simulink library "xrbsComm_r3"  (Simulink 5.1)
libraries: xbsIndex_r3 x775, xrbsComm_r3 x1
(part 1 of 6)
settings Model: Creator=singhj  LastModifiedBy=annr  ProdHWDeviceType=Microprocessor

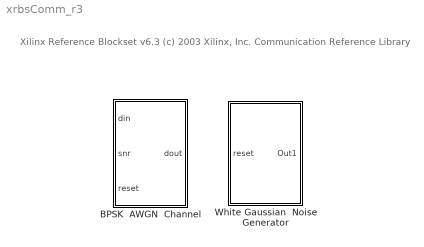
== system xrbsComm_r3 ==
  note: Xilinx Reference Blockset v6.3
      | (c) 2003  Xilinx, Inc.
      |
      | Communication Reference Library
  BPSK  AWGN  Channel : Subsystem  mask(BPSK AWGN Channel){seed=510}
      mask prompts: seed "Decimal Seed Value"
      mask help: Binary Phase Shift Keying Additive White Gaussian Noise Channel. Adds scaled white Gaussian nose to an input signal.
      mask init:
      | [bg,fg] = xlcmap('XBlock',0);
      | iPos = get_param(gcb,'Position');
      | iWidth=iPos(3)-iPos(1); iHeight=iPos(4)-iPos(2);
      | iCx=iWidth/2;
      | iCy=iHeight/2;
      | [logoX, logoY] = xlogo(iPos);
      mask Help:
      | web(xldoclink('BPSK
      | AWGN
      | Channel'));
      mask Display:
      | patch([0 iWidth iWidth 0],[0 0 iHeight iHeight] , bg);
      | patch(logoX,logoY , fg);
      | port_label('input',1,'din');
      | port_label('input',2,'snr');
      | port_label('input',3,'reset');
      | port_label('output',1,'dout');
      | plot([0 0 iWidth iWidth 0], [0 iHeight iHeight 0 0]);
  White Gaussian  Noise Generator : Subsystem  mask(White Gaussian Noise Generator){seed=512}
      mask help: White Gaussian Noise Generator. Generates white Gaussian noise using a combination of the Box-Muller algorithm and the central limit theorem.
      mask init:
      | old_seed = rand('seed');
      | rand('seed',seed);
      | init1 = [dec2hex(floor(rand*16)) dec2hex(floor(rand*16)) dec2hex(floor(rand*16)) ...
      | 		dec2hex(floor(rand*16)) dec2hex(floor(rand*16)) dec2hex(floor(rand*16)) ...
      | 		dec2hex(floor(rand*16)) dec2hex(floor(rand*16)) dec2hex(floor(rand*16)) ...
      | 		dec2hex(floor(rand*16)) dec2hex(floor(rand*16)) dec2hex(floor(rand*16))];
      | seed1 = hex2dec(init1);
      | init2 = [dec2hex(floor(rand*16)) dec2hex(floor(rand*16)) dec2hex(floor(rand*16)) ...
      | 		dec2hex(floor(rand*16)) dec2hex(floor(rand*16)) dec2hex(floor(rand*16)) ...
      | 		dec2hex(floor(rand*16)) dec2hex(floor(rand*16)) dec2hex(floor(rand*16)) ...
      | 		dec2hex(floor(rand*16)) dec2hex(floor(rand*16)) dec2hex(floor(rand*16))];
      | seed2 = hex2dec(init2);
      | init3 = [dec2hex(floor(rand*16)) dec2hex(floor(rand*16)) dec2hex(floor(rand*16)) ...
      | 		dec2hex(floor(rand*16)) dec2hex(floor(rand*16)) dec2hex(floor(rand*16)) ...
      | 		dec2hex(floor(rand*16)) dec2hex(floor(rand*16)) dec2hex(floor(rand*16)) ...
      | 		dec2hex(floor(rand*16)) dec2hex(floor(rand*16)) dec2hex(floor(rand*16))];
      | seed3 = hex2dec(init3);
      | init4 = [dec2hex(floor(rand*16)) dec2hex(floor(rand*16)) dec2hex(floor(rand*16)) ...
      | 		dec2hex(floor(rand*16)) dec2hex(floor(rand*16)) dec2hex(floor(rand*16)) ...
      | 		dec2hex(floor(rand*16)) dec2hex(floor(rand*16)) dec2hex(floor(rand*16)) ...
      | 		dec2hex(floor(rand*16)) dec2hex(floor(rand*16)) dec2hex(floor(rand*16))];
      | seed4 = hex2dec(init4);
      | rand('seed',old_seed);
      | 
      | 
      | [bg,fg] = xlcmap('XBlock',0);
      | iPos = get_param(gcb,'Position');
      | iWidth=iPos(3)-iPos(1); iHeight=iPos(4)-iPos(2);
      | iCx=iWidth/2;
      | iCy=iHeight/2;
      | [logoX, logoY] = xlogo(iPos);
      mask Help: web(xlhtmldoclink('White Gaussian  Noise Generator'));
      mask Display:
      | patch([0 iWidth iWidth 0],[0 0 iHeight iHeight] , bg);
      | patch(logoX,logoY , fg);
      | port_label('input',1,'reset');
      | port_label('output',1,'noise');
      | plot([0 0 iWidth iWidth 0], [0 iHeight iHeight 0 0]);

== system xrbsComm_r3/BPSK  AWGN  Channel ==
  note: The WGNG block generates a probability density function (PDF) that is Gaussian to within .2% for
      | 4.8 standard deviations from the mean.  The PDF is scaled based on the value of the signal to noise
      | ratio to achieve the desired noise variance.  The SNR input is defined as (Eb/No) in dB for uncoded BPSK
      | with unit symbol energy (Es = 1).  If the SNR input is of type UFix8_4, the valid range is from 0.0 to 15.9375
      | in steps of 0.0625dB.  To use the AWGN in a system with coding and/or to use the core with different
      | modulation formats, it is necessary to adjust the SNR value to accommodate the difference in spectral
      | efficiency.  If we have BPSK modulation with rate 1/2 coding and keep Es = 1and No constant, then Eb = 2
      | and Eb/No = SNR + 3 dB.  If we have uncoded QPSK modulation with I = +/-1 and Q = +/-1 and add
      | independent noise sequences, then each channel looks like and independent BPSK channel and the
      | Eb/No = SNR.  If we then add rate 1/2 coding to the QPSK case, we have Eb/No = SNR + 3 dB.
      |
      | For more information see:
      |
      | [1] A. Ghazel, E. Boutillon, J. L. Danger, G. Gulak and H. Laamari, "Design and Performance Analysis of a
      | High Speed AWGN Communication Channel Emulator" IEEE PACRIM Conference, Victoria, B. C., Aug.
      | 2001.
      | [2] Xilinx Data Sheet: Additive White Gaussian Noise (AWGN) Core v1.0, Xilinx, Inc. October 2002
  din : Inport
  snr : Inport  Port=2
  reset : Inport  Port=3
  AddSub : xbsIndex_r3/AddSub  mode=Addition  precision=Full  arith_type=Unsigned  n_bits=8  bin_pt=2  quantization=Truncate  overflow=Wrap  latency=1  explicit_period=off  period=1  use_carryin=off  use_carryout=off  en=off  dbl_ovrd=off  show_param=off  use_core=on  pipeline=off  use_rpm=off  gen_core=on
      settings: xl_area=[0, 0, 0, 0, 0, 0, 0]
  Constant1 : xbsIndex_r3/Constant  const=1  arith_type="Signed  (2's comp)"  n_bits=2  bin_pt=0  explicit_period=off  period=1  dbl_ovrd=off
  Constant2 : xbsIndex_r3/Constant  const=-1  arith_type="Signed  (2's comp)"  n_bits=2  bin_pt=0  explicit_period=off  period=1  dbl_ovrd=off
  Convert : xbsIndex_r3/Convert  arith_type="Signed  (2's comp)"  n_bits=16  bin_pt=11  quantization="Round  (unbiased: +/- Inf)"  overflow=Wrap  latency=2  explicit_period=off  period=1  dbl_ovrd=off  show_param=off  inserted_by_tool=off
      settings: xl_area=[0, 0, 0, 0, 0, 0, 0]
  Delay : xbsIndex_r3/Delay  latency=14  reg_retiming=off  explicit_period=off  period=1  en=off  accept_only_valid=off  init_zero=on  dbl_ovrd=off  show_param=off
      settings: xl_area=[0, 0, 0, 0, 0, 0, 0]
  Input  Conversion : Subsystem
  Mult : xbsIndex_r3/Mult  precision=Full  arith_type="Signed  (2's comp)"  n_bits=8  bin_pt=2  quantization=Truncate  overflow=Wrap  latency=2  explicit_period=off  period=1  en=off  dbl_ovrd=off  show_param=off  mult_type=Parallel  oversample=2  use_embedded=on  pipeline=off  use_rpm=off  placement_style=Rectangular Shape  gen_core=on
      settings: xl_area=[0, 0, 0, 0, 0, 0, 0]
  Mux : xbsIndex_r3/Mux  inputs=2  precision=Full  arith_type="Signed  (2's comp)"  n_bits=8  bin_pt=2  quantization=Truncate  overflow=Wrap  latency=0  explicit_period=off  period=-1  en=off  dbl_ovrd=off  show_param=off  mux_type=off  use_rpm=off  gen_core=on
      settings: xl_area=[0, 0, 0, 0, 0, 0, 0]
  ROM : xbsIndex_r3/ROM  depth=256  initVector=((2*10.^(0.1*(([0:255]/10) - 0.6*floor([0:255]/16) ))).^(-0.5))*1.0023  arith_type=Unsigned  n_bits=15  bin_pt=15  latency=1  init_zero=on  explicit_period=off  period=1  rst=off  init_reg=0  en=off  dbl_ovrd=off  show_param=off  distributed_mem=off  use_rpm=off  gen_core=on
      settings: xl_area=[0, 0, 0, 0, 0, 0, 0]
  White Gaussian  Noise Generator : xrbsComm_r3/White Gaussian  Noise Generator  seed=512
  dout : Outport
  wires:
  reset/1 -> White Gaussian  Noise Generator/1
  Delay/1 -> AddSub/1
  Convert/1 -> AddSub/2
  White Gaussian  Noise Generator/1 -> Mult/2
  din/1 -> Mux/1
  snr/1 -> Input  Conversion/1(" ")
  Mult/1 -> Convert/1
  ROM/1 -> Mult/1
  AddSub/1 -> dout/1
  Input  Conversion/1(conv) -> ROM/1
  Constant1/1 -> Mux/2
  Constant2/1 -> Mux/3
  Mux/1 -> Delay/1

== system xrbsComm_r3/White Gaussian  Noise Generator ==
  note: The WGNG generates white Gaussian noise using a combination of the Box-Muller algorithm and the Central Limit Theorem
      | following the general approach described in [1].   The Box-Muller algorithm generates a unit normal random variable via a
      | transformation of two independent random variables that are uniformly distributed over [0,1].  This is accomplished by storing
      | Box-Muller function values in ROMs and addressing them with uniform random variables.  The uniform random variables are
      | produced by multiple-bit leap-forward LFSRs.  A standard LFSR generates one output per clock cycle.  K-bit leap-forward LFSRs
      | are able to generate k outputs in a single cycle.  For example, a 4-bit leap-forward LFSR outputs a discrete uniform random
      | variable between 0 and 15.  A portion of the 48-bit block parameter seed initializes each LFSR allowing customization.  The
      | outputs of four parallel Box-Muller subsystems are averaged to obtain a probability density function (PDF) that is Gaussian.
      | The overall latency of the WGNG is 10 clock cycles.  The output port noise is a 12 bit signed number with 7 bits after the binary
      | point.
      |
      | [1] A. Ghazel, E. Boutillon, J. L. Danger, G. Gulak and H. Laamari, "Design and Performance Analysis of a
      | High Speed AWGN Communication Channel Emulator" IEEE PACRIM Conference, Victoria, B. C., Aug. 2001.
  " reset" : Inport
  AddSub : xbsIndex_r3/AddSub  mode=Addition  precision=Full  arith_type=Unsigned  n_bits=8  bin_pt=2  quantization=Truncate  overflow=Wrap  latency=1  explicit_period=off  period=1  use_carryin=off  use_carryout=off  en=off  dbl_ovrd=off  show_param=off  use_core=on  pipeline=off  use_rpm=off  gen_core=on
      settings: xl_area=[0, 0, 0, 0, 0, 0, 0]
  AddSub1 : xbsIndex_r3/AddSub  mode=Addition  precision=Full  arith_type=Unsigned  n_bits=8  bin_pt=2  quantization=Truncate  overflow=Wrap  latency=1  explicit_period=off  period=1  use_carryin=off  use_carryout=off  en=off  dbl_ovrd=off  show_param=off  use_core=on  pipeline=off  use_rpm=off  gen_core=on
      settings: xl_area=[0, 0, 0, 0, 0, 0, 0]
  AddSub2 : xbsIndex_r3/AddSub  mode=Addition  precision=Full  arith_type=Unsigned  n_bits=8  bin_pt=2  quantization=Truncate  overflow=Wrap  latency=1  explicit_period=off  period=1  use_carryin=off  use_carryout=off  en=off  dbl_ovrd=off  show_param=off  use_core=on  pipeline=off  use_rpm=off  gen_core=on
      settings: xl_area=[0, 0, 0, 0, 0, 0, 0]
  Box-Muller1 : Subsystem  mask(Box-Muller){f_init1=bitget(seed1, 17:-1:1), f_init2=bitget(seed1, 25:-1:1), f_init3=bitget(seed1, 29:-1:1), f_init4=bitget(seed1, 31:-1:1), f_init5=bitget(seed1, 41:-1:1), g_init=bitget(seed1, 47:-1:1)}
      mask prompts: f_init1 "f_init1(17:1)"; f_init2 "f_init2(25:1)"; f_init3 "f_init3(29:1)"; f_init4 "f_init4(31:1)"; f_init5 "f_init5(41:1)"; g_init "g_init(47:1)"
  Box-Muller2 : Subsystem  mask(Box-Muller){f_init1=bitget(seed2, 17:-1:1), f_init2=bitget(seed2, 25:-1:1), f_init3=bitget(seed2, 29:-1:1), f_init4=bitget(seed2, 31:-1:1), f_init5=bitget(seed2, 41:-1:1), g_init=bitget(seed2, 47:-1:1)}
      mask prompts: f_init1 "f_init1(17:1)"; f_init2 "f_init2(25:1)"; f_init3 "f_init3(29:1)"; f_init4 "f_init4(31:1)"; f_init5 "f_init5(41:1)"; g_init "g_init(47:1)"
  Box-Muller3 : Subsystem  mask(Box-Muller){f_init1=bitget(seed3, 17:-1:1), f_init2=bitget(seed3, 25:-1:1), f_init3=bitget(seed3, 29:-1:1), f_init4=bitget(seed3, 31:-1:1), f_init5=bitget(seed3, 41:-1:1), g_init=bitget(seed3,47:-1:1)}
      mask prompts: f_init1 "f_init1(17:1)"; f_init2 "f_init2(25:1)"; f_init3 "f_init3(29:1)"; f_init4 "f_init4(31:1)"; f_init5 "f_init5(41:1)"; g_init "g_init(47:1)"
  Box-Muller4 : Subsystem  mask(Box-Muller){f_init1=bitget(seed4, 17:-1:1), f_init2=bitget(seed4, 25:-1:1), f_init3=bitget(seed4, 29:-1:1), f_init4=bitget(seed4, 31:-1:1), f_init5=bitget(seed4, 41:-1:1), g_init=bitget(seed4, 47:-1:1)}
      mask prompts: f_init1 "f_init1(17:1)"; f_init2 "f_init2(25:1)"; f_init3 "f_init3(29:1)"; f_init4 "f_init4(31:1)"; f_init5 "f_init5(41:1)"; g_init "g_init(47:1)"
  Reinterpret : xbsIndex_r3/Reinterpret  force_arith_type=off  arith_type=Unsigned  force_bin_pt=on  bin_pt=7  force_valid=on
  Out1 : Outport
  wires:
  " reset"/1 -> Box-Muller3/1(reset), Box-Muller4/1(reset), Box-Muller2/1(reset), Box-Muller1/1(" reset")
  Reinterpret/1 -> Out1/1
  Box-Muller4/1(bm) -> AddSub1/2
  Box-Muller3/1(bm) -> AddSub1/1
  Box-Muller2/1(bm) -> AddSub/2
  Box-Muller1/1(bm) -> AddSub/1
  AddSub2/1 -> Reinterpret/1
  AddSub1/1 -> AddSub2/2
  AddSub/1 -> AddSub2/1

== system xrbsComm_r3/BPSK  AWGN  Channel/Input  Conversion ==
  " " : Inport
  AddSub1 : xbsIndex_r3/AddSub  mode=Addition  precision=User Defined  arith_type=Unsigned  n_bits=8  bin_pt=0  quantization=Truncate  overflow=Wrap  latency=0  explicit_period=off  period=1  en=off  dbl_ovrd=off  use_core=on  gen_core=on  pipeline=off  use_rpm=off
      settings: xl_area=[0, 0, 0, 0, 0, 0, 0]
  CMult : xbsIndex_r3/CMult  const=16  const_n_bits=5  const_bin_pt=0  precision=Full  arith_type="Signed  (2's comp)"  n_bits=8  bin_pt=6  quantization="Round  (unbiased: +/- Inf)"  overflow=Wrap  mult_type=Parallel  mem_type=Distributed RAM  pipeline=off  latency=0  explicit_period=off  period=1  en=off  dbl_ovrd=off  oversample=2  gen_core=on  use_rpm=off  placement_style=Rectangular Shape
      settings: xl_area=[0, 0, 0, 0, 0, 0, 0]
  CMult1 : xbsIndex_r3/CMult  const=10  const_n_bits=4  const_bin_pt=0  precision=Full  arith_type="Signed  (2's comp)"  n_bits=8  bin_pt=6  quantization="Round  (unbiased: +/- Inf)"  overflow=Wrap  mult_type=Parallel  mem_type=Distributed RAM  pipeline=off  latency=0  explicit_period=off  period=1  en=off  dbl_ovrd=off  oversample=2  gen_core=on  use_rpm=off  placement_style=Rectangular Shape
      settings: xl_area=[0, 0, 0, 0, 0, 0, 0]
  Shift : xbsIndex_r3/Shift  shift_dir=Right  shift_bits=4  precision=User Defined  arith_type=Unsigned  n_bits=4  bin_pt=0  quantization=Truncate  overflow=Wrap  latency=0  explicit_period=off  period=1  en=off  dbl_ovrd=off
      settings: xl_area=[0, 0, 0, 0, 0, 0, 0]
  Slice : xbsIndex_r3/Slice  mode=Upper Bit Location + Width  nbits=4  bit1=0  base1=MSB of Input  bit0=0  base0=LSB of Input  boolean_output=off  explicit_period=off  period=1  dbl_ovrd=off
  Slice1 : xbsIndex_r3/Slice  mode=Lower Bit Location + Width  nbits=4  bit1=0  base1=MSB of Input  bit0=0  base0=LSB of Input  boolean_output=off  explicit_period=off  period=1  dbl_ovrd=off
  conv : Outport
  wires:
  Slice/1 -> CMult/1
  Slice1/1 -> CMult1/1
  AddSub1/1 -> conv/1
  CMult/1 -> AddSub1/1
  " "/1 -> Slice/1, Slice1/1
  CMult1/1 -> Shift/1
  Shift/1 -> AddSub1/2

== system xrbsComm_r3/White Gaussian  Noise Generator/Box-Muller1 ==
  " reset" : Inport
  Convert : xbsIndex_r3/Convert  arith_type="Signed  (2's comp)"  n_bits=10  bin_pt=6  quantization="Round  (unbiased: +/- Inf)"  overflow=Wrap  latency=2  explicit_period=off  period=1  dbl_ovrd=off  inserted_by_tool=off
      settings: xl_area=[0, 0, 0, 0, 0, 0, 0]
  Mult : xbsIndex_r3/Mult  precision=Full  arith_type="Signed  (2's comp)"  n_bits=20  bin_pt=0  quantization="Round  (unbiased: +/- Inf)"  overflow=Wrap  mult_type=Parallel  use_embedded=on  pipeline=on  latency=2  explicit_period=off  period=1  en=off  dbl_ovrd=off  oversample=2  gen_core=on  use_rpm=off  placement_style=Rectangular Shape
      settings: xl_area=[0, 0, 0, 0, 0, 0, 0]
  f : Subsystem  mask(f_rom){init1=f_init1, init2=f_init2, init3=f_init3, init4=f_init4, init5=f_init5}
      mask prompts: init1 "init1(17:1)"; init2 "init2(25:1)"; init3 "init3(29:1)"; init4 "init4(31:1)"; init5 "init5(41:1)"
  g : Subsystem  mask{init=g_init}
      mask prompts: init "g_init(47:1)"
  bm : Outport
  wires:
  g/1(g(s')) -> Mult/2
  f/1(f(s')) -> Mult/1
  Mult/1 -> Convert/1
  Convert/1 -> bm/1
  " reset"/1 -> f/1("reset "), g/1(reset)

== system xrbsComm_r3/White Gaussian  Noise Generator/Box-Muller2 ==
  reset : Inport
  Convert : xbsIndex_r3/Convert  arith_type="Signed  (2's comp)"  n_bits=10  bin_pt=6  quantization="Round  (unbiased: +/- Inf)"  overflow=Wrap  latency=2  explicit_period=off  period=1  dbl_ovrd=off  inserted_by_tool=off
      settings: xl_area=[0, 0, 0, 0, 0, 0, 0]
  Mult : xbsIndex_r3/Mult  precision=Full  arith_type="Signed  (2's comp)"  n_bits=20  bin_pt=0  quantization="Round  (unbiased: +/- Inf)"  overflow=Wrap  mult_type=Parallel  use_embedded=on  pipeline=on  latency=2  explicit_period=off  period=1  en=off  dbl_ovrd=off  oversample=2  gen_core=on  use_rpm=off  placement_style=Rectangular Shape
      settings: xl_area=[0, 0, 0, 0, 0, 0, 0]
  fr1 : Subsystem  mask(f_rom){init1=f_init1, init2=f_init2, init3=f_init3, init4=f_init4, init5=f_init5}
      mask prompts: init1 "init1(17:1)"; init2 "init2(25:1)"; init3 "init3(29:1)"; init4 "init4(31:1)"; init5 "init5(41:1)"
  g2 : Subsystem  mask{init=g_init}
      mask prompts: init "g_init(47:1)"
  bm : Outport
  wires:
  g2/1(g(s')) -> Mult/2
  Mult/1 -> Convert/1
  Convert/1 -> bm/1
  reset/1 -> fr1/1(reset), g2/1(reset)
  fr1/1(f(s')) -> Mult/1

== system xrbsComm_r3/White Gaussian  Noise Generator/Box-Muller3 ==
  reset : Inport
  Convert : xbsIndex_r3/Convert  arith_type="Signed  (2's comp)"  n_bits=10  bin_pt=6  quantization="Round  (unbiased: +/- Inf)"  overflow=Wrap  latency=2  explicit_period=off  period=1  dbl_ovrd=off  inserted_by_tool=off
      settings: xl_area=[0, 0, 0, 0, 0, 0, 0]
  Mult : xbsIndex_r3/Mult  precision=Full  arith_type="Signed  (2's comp)"  n_bits=20  bin_pt=0  quantization="Round  (unbiased: +/- Inf)"  overflow=Wrap  mult_type=Parallel  use_embedded=on  pipeline=on  latency=2  explicit_period=off  period=1  en=off  dbl_ovrd=off  oversample=2  gen_core=on  use_rpm=off  placement_style=Rectangular Shape
      settings: xl_area=[0, 0, 0, 0, 0, 0, 0]
  fr1 : Subsystem  mask(f_rom){init1=f_init1, init2=f_init2, init3=f_init3, init4=f_init4, init5=f_init5}
      mask prompts: init1 "init1(17:1)"; init2 "init2(25:1)"; init3 "init3(29:1)"; init4 "init4(31:1)"; init5 "init5(41:1)"
  g2 : Subsystem  mask{init=g_init}
      mask prompts: init "g_init(47:1)"
  bm : Outport
  wires:
  g2/1(g(s')) -> Mult/2
  fr1/1(f(s')) -> Mult/1
  Mult/1 -> Convert/1
  Convert/1 -> bm/1
  reset/1 -> fr1/1(reset), g2/1(reset)

== system xrbsComm_r3/White Gaussian  Noise Generator/Box-Muller4 ==
  reset : Inport
  Convert : xbsIndex_r3/Convert  arith_type="Signed  (2's comp)"  n_bits=10  bin_pt=6  quantization="Round  (unbiased: +/- Inf)"  overflow=Wrap  latency=2  explicit_period=off  period=1  dbl_ovrd=off  inserted_by_tool=off
      settings: xl_area=[0, 0, 0, 0, 0, 0, 0]
  Mult : xbsIndex_r3/Mult  precision=Full  arith_type="Signed  (2's comp)"  n_bits=20  bin_pt=0  quantization="Round  (unbiased: +/- Inf)"  overflow=Wrap  mult_type=Parallel  use_embedded=on  pipeline=on  latency=2  explicit_period=off  period=1  en=off  dbl_ovrd=off  oversample=2  gen_core=on  use_rpm=off  placement_style=Rectangular Shape
      settings: xl_area=[0, 0, 0, 0, 0, 0, 0]
  fr1 : Subsystem  mask(f_rom){init1=f_init1, init2=f_init2, init3=f_init3, init4=f_init4, init5=f_init5}
      mask prompts: init1 "init1(17:1)"; init2 "init2(25:1)"; init3 "init3(29:1)"; init4 "init4(31:1)"; init5 "init5(41:1)"
  g2 : Subsystem  mask{init=g_init}
      mask prompts: init "g_init(47:1)"
  bm : Outport
  wires:
  reset/1 -> g2/1(reset), fr1/1(reset)
  g2/1(g(s')) -> Mult/2
  fr1/1(f(s')) -> Mult/1
  Mult/1 -> Convert/1
  Convert/1 -> bm/1

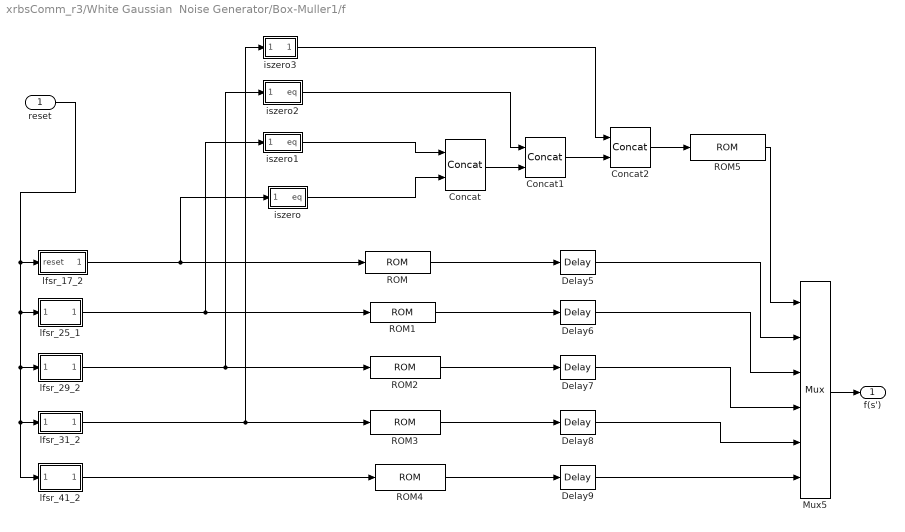
== system xrbsComm_r3/White Gaussian  Noise Generator/Box-Muller1/f ==
  "reset " : Inport
  Concat : xbsIndex_r3/Concat  explicit_period=off  period=1  dbl_ovrd=off
  Concat1 : xbsIndex_r3/Concat  explicit_period=off  period=1  dbl_ovrd=off
  Concat2 : xbsIndex_r3/Concat  explicit_period=off  period=1  dbl_ovrd=off
  Delay{5..9} (5 alike) : xbsIndex_r3/Delay  latency=2  explicit_period=off  period=1  en=off  accept_only_valid=off  init_zero=on  dbl_ovrd=off
      settings: xl_area=[0, 0, 0, 0, 0, 0, 0]
  Mux5 : xbsIndex_r3/Mux  inputs=5  precision=Full  arith_type="Signed  (2's comp)"  n_bits=10  bin_pt=0  quantization="Round  (unbiased: +/- Inf)"  overflow=Wrap  latency=1  mux_type=off  explicit_period=off  period=1  en=off  dbl_ovrd=off  gen_core=on  use_rpm=off
      settings: xl_area=[0, 0, 0, 0, 0, 0, 0]
  ROM : xbsIndex_r3/ROM  depth=16  initVector=sqrt(-log( ((0:15)+0.51)'*(2.^(-1.*4)) ))  arith_type=Unsigned  n_bits=9  bin_pt=7  latency=1  distributed_mem=on  init_zero=on  explicit_period=off  period=1  en=off  dbl_ovrd=off  gen_core=on  use_rpm=off
      settings: xl_area=[0, 0, 0, 0, 0, 0, 0]
  ROM1 : xbsIndex_r3/ROM  depth=16  initVector=sqrt(-log( ((0:15)+0.51)'*(2.^(-2.*4)) ))  arith_type=Unsigned  n_bits=9  bin_pt=7  latency=1  distributed_mem=on  init_zero=on  explicit_period=off  period=1  en=off  dbl_ovrd=off  gen_core=on  use_rpm=off
      settings: xl_area=[0, 0, 0, 0, 0, 0, 0]
  ROM2 : xbsIndex_r3/ROM  depth=16  initVector=sqrt(-log( ((0:15)+0.51)'*(2.^(-3.*4)) ))  arith_type=Unsigned  n_bits=9  bin_pt=7  latency=1  distributed_mem=on  init_zero=on  explicit_period=off  period=1  en=off  dbl_ovrd=off  gen_core=on  use_rpm=off
      settings: xl_area=[0, 0, 0, 0, 0, 0, 0]
  ROM3 : xbsIndex_r3/ROM  depth=16  initVector=sqrt(-log( ((0:15)+0.51)'*(2.^(-4.*4)) ))  arith_type=Unsigned  n_bits=9  bin_pt=7  latency=1  distributed_mem=on  init_zero=on  explicit_period=off  period=1  en=off  dbl_ovrd=off  gen_core=on  use_rpm=off
      settings: xl_area=[0, 0, 0, 0, 0, 0, 0]
  ROM4 : xbsIndex_r3/ROM  depth=16  initVector=sqrt(-log( ((0:15)+0.51)'*(2.^(-5.*4)) ))  arith_type=Unsigned  n_bits=9  bin_pt=7  latency=1  distributed_mem=on  init_zero=on  explicit_period=off  period=1  en=off  dbl_ovrd=off  gen_core=on  use_rpm=off
      settings: xl_area=[0, 0, 0, 0, 0, 0, 0]
  ROM5 : xbsIndex_r3/ROM  depth=16  initVector=[0 1 0 2 0 1 0 3 0 1 0 2 0 1 0 4]  arith_type=Unsigned  n_bits=3  bin_pt=0  latency=2  distributed_mem=off  init_zero=on  explicit_period=off  period=1  en=off  dbl_ovrd=off  gen_core=on  use_rpm=off
      settings: xl_area=[0, 0, 0, 0, 0, 0, 0]
  iszero : Subsystem
  iszero1 : Subsystem
  iszero2 : Subsystem
  iszero3 : Subsystem
  lfsr_17_2 : Subsystem  mask(lfsr_17){init=init1}
      mask prompts: init "init(17:1)"
  lfsr_25_1 : Subsystem  mask(lfsr_25){init=init2}
      mask prompts: init "init(25:1)"
  lfsr_29_2 : Subsystem  mask(lfsr_29){init=init3}
      mask prompts: init "init(29:1)"
  lfsr_31_2 : Subsystem  mask(lfsr_31){init=init4}
      mask prompts: init "init(31:1)"
  lfsr_41_2 : Subsystem  mask(lfsr_41){init=init5}
      mask prompts: init "init(41:1)"
  f(s') : Outport
  wires:
  lfsr_17_2/1(" ") -> ROM/1, iszero/1(" ")
  lfsr_25_1/1(" ") -> ROM1/1, iszero1/1(" ")
  lfsr_29_2/1(" ") -> ROM2/1, iszero2/1(" ")
  lfsr_31_2/1(" ") -> iszero3/1(" "), ROM3/1
  lfsr_41_2/1(" ") -> ROM4/1
  Concat2/1 -> ROM5/1
  ROM5/1 -> Mux5/1
  Concat/1 -> Concat1/2
  Concat1/1 -> Concat2/2
  Mux5/1 -> f(s')/1
  ROM/1 -> Delay5/1
  ROM1/1 -> Delay6/1
  ROM2/1 -> Delay7/1
  ROM3/1 -> Delay8/1
  ROM4/1 -> Delay9/1
  iszero/1(eq) -> Concat/2
  iszero1/1(eq) -> Concat/1
  iszero2/1(eq) -> Concat1/1
  iszero3/1(eq) -> Concat2/1
  Delay5/1 -> Mux5/2
  Delay6/1 -> Mux5/3
  Delay7/1 -> Mux5/4
  Delay8/1 -> Mux5/5
  Delay9/1 -> Mux5/6
  "reset "/1 -> lfsr_25_1/1(" reset"), lfsr_41_2/1(reset), lfsr_31_2/1(reset), lfsr_29_2/1(reset), lfsr_17_2/1(reset)

== system xrbsComm_r3/White Gaussian  Noise Generator/Box-Muller1/g ==
  reset : Inport
  Delay : xbsIndex_r3/Delay  latency=3  explicit_period=off  period=1  en=off  accept_only_valid=off  init_zero=on  dbl_ovrd=off
      settings: xl_area=[0, 0, 0, 0, 0, 0, 0]
  ROM : xbsIndex_r3/ROM  depth=256  initVector=sqrt(2) * cos(pi*((0:255) + 0.5)*2^(-8))  arith_type="Signed  (2's comp)"  n_bits=10  bin_pt=8  latency=1  distributed_mem=off  init_zero=on  explicit_period=off  period=1  en=off  dbl_ovrd=off  gen_core=on  use_rpm=off
      settings: xl_area=[0, 0, 0, 0, 0, 0, 0]
  lfsr_47_5 : Subsystem  mask(lfsr_47){init=init}
      mask prompts: init "init(47:1)"
  g(s') : Outport
  wires:
  ROM/1 -> Delay/1
  lfsr_47_5/1(" ") -> ROM/1
  Delay/1 -> g(s')/1
  reset/1 -> lfsr_47_5/1(reset)

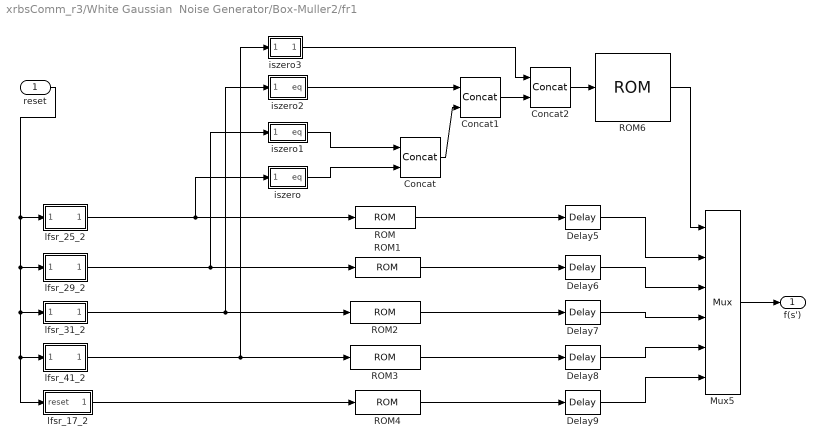
== system xrbsComm_r3/White Gaussian  Noise Generator/Box-Muller2/fr1 ==
  reset : Inport
  Concat : xbsIndex_r3/Concat  explicit_period=off  period=1  dbl_ovrd=off
  Concat1 : xbsIndex_r3/Concat  explicit_period=off  period=1  dbl_ovrd=off
  Concat2 : xbsIndex_r3/Concat  explicit_period=off  period=1  dbl_ovrd=off
  Delay{5..9} (5 alike) : xbsIndex_r3/Delay  latency=2  explicit_period=off  period=1  en=off  accept_only_valid=off  init_zero=on  dbl_ovrd=off
      settings: xl_area=[0, 0, 0, 0, 0, 0, 0]
  Mux5 : xbsIndex_r3/Mux  inputs=5  precision=Full  arith_type="Signed  (2's comp)"  n_bits=10  bin_pt=0  quantization="Round  (unbiased: +/- Inf)"  overflow=Wrap  latency=1  mux_type=off  explicit_period=off  period=1  en=off  dbl_ovrd=off  gen_core=on  use_rpm=off
      settings: xl_area=[0, 0, 0, 0, 0, 0, 0]
  ROM : xbsIndex_r3/ROM  depth=16  initVector=sqrt(-log( ((0:15)+0.51)'*(2.^(-1.*4)) ))  arith_type=Unsigned  n_bits=9  bin_pt=7  latency=1  distributed_mem=on  init_zero=on  explicit_period=off  period=1  en=off  dbl_ovrd=off  gen_core=on  use_rpm=off
      settings: xl_area=[0, 0, 0, 0, 0, 0, 0]
  ROM1 : xbsIndex_r3/ROM  depth=16  initVector=sqrt(-log( ((0:15)+0.51)'*(2.^(-2.*4)) ))  arith_type=Unsigned  n_bits=9  bin_pt=7  latency=1  distributed_mem=on  init_zero=on  explicit_period=off  period=1  en=off  dbl_ovrd=off  gen_core=on  use_rpm=off
      settings: xl_area=[0, 0, 0, 0, 0, 0, 0]
  ROM2 : xbsIndex_r3/ROM  depth=16  initVector=sqrt(-log( ((0:15)+0.51)'*(2.^(-3.*4)) ))  arith_type=Unsigned  n_bits=9  bin_pt=7  latency=1  distributed_mem=on  init_zero=on  explicit_period=off  period=1  en=off  dbl_ovrd=off  gen_core=on  use_rpm=off
      settings: xl_area=[0, 0, 0, 0, 0, 0, 0]
  ROM3 : xbsIndex_r3/ROM  depth=16  initVector=sqrt(-log( ((0:15)+0.51)'*(2.^(-4.*4)) ))  arith_type=Unsigned  n_bits=9  bin_pt=7  latency=1  distributed_mem=on  init_zero=on  explicit_period=off  period=1  en=off  dbl_ovrd=off  gen_core=on  use_rpm=off
      settings: xl_area=[0, 0, 0, 0, 0, 0, 0]
  ROM4 : xbsIndex_r3/ROM  depth=16  initVector=sqrt(-log( ((0:15)+0.51)'*(2.^(-5.*4)) ))  arith_type=Unsigned  n_bits=9  bin_pt=7  latency=1  distributed_mem=on  init_zero=on  explicit_period=off  period=1  en=off  dbl_ovrd=off  gen_core=on  use_rpm=off
      settings: xl_area=[0, 0, 0, 0, 0, 0, 0]
  ROM6 : xbsIndex_r3/ROM  depth=16  initVector=[0 1 0 2 0 1 0 3 0 1 0 2 0 1 0 4]  arith_type=Unsigned  n_bits=3  bin_pt=0  latency=2  distributed_mem=off  init_zero=on  explicit_period=off  period=1  en=off  dbl_ovrd=off  gen_core=on  use_rpm=off
      settings: xl_area=[0, 0, 0, 0, 0, 0, 0]
  iszero : Subsystem
  iszero1 : Subsystem
  iszero2 : Subsystem
  iszero3 : Subsystem
  lfsr_17_2 : Subsystem  mask(lfsr_17){init=init1}
      mask prompts: init "init(17:1)"
  lfsr_25_2 : Subsystem  mask(lfsr_25){init=init2}
      mask prompts: init "init(25:1)"
  lfsr_29_2 : Subsystem  mask(lfsr_29){init=init3}
      mask prompts: init "init(29:1)"
  lfsr_31_2 : Subsystem  mask(lfsr_31){init=init4}
      mask prompts: init "init(31:1)"
  lfsr_41_2 : Subsystem  mask(lfsr_41){init=init5}
      mask prompts: init "init(41:1)"
  f(s') : Outport
  wires:
  Delay9/1 -> Mux5/6
  Delay8/1 -> Mux5/5
  Delay7/1 -> Mux5/4
  Delay6/1 -> Mux5/3
  Delay5/1 -> Mux5/2
  iszero/1(eq) -> Concat/2
  lfsr_25_2/1(" ") -> iszero/1(" "), ROM/1
  lfsr_29_2/1(" ") -> ROM1/1, iszero1/1(" ")
  lfsr_31_2/1(" ") -> iszero2/1(" "), ROM2/1
  lfsr_41_2/1(" ") -> ROM3/1, iszero3/1(" ")
  lfsr_17_2/1(" ") -> ROM4/1
  Concat/1 -> Concat1/2
  Concat1/1 -> Concat2/2
  ROM/1 -> Delay5/1
  ROM1/1 -> Delay6/1
  ROM4/1 -> Delay9/1
  ROM6/1 -> Mux5/1
  iszero1/1(eq) -> Concat/1
  Concat2/1 -> ROM6/1
  iszero2/1(eq) -> Concat1/1
  iszero3/1(eq) -> Concat2/1
  ROM2/1 -> Delay7/1
  ROM3/1 -> Delay8/1
  Mux5/1 -> f(s')/1
  reset/1 -> lfsr_25_2/1(" reset"), lfsr_29_2/1(reset), lfsr_31_2/1(reset), lfsr_17_2/1(reset), lfsr_41_2/1(reset)

== system xrbsComm_r3/White Gaussian  Noise Generator/Box-Muller2/g2 ==
  reset : Inport
  Delay : xbsIndex_r3/Delay  latency=3  explicit_period=off  period=1  en=off  accept_only_valid=off  init_zero=on  dbl_ovrd=off
      settings: xl_area=[0, 0, 0, 0, 0, 0, 0]
  ROM : xbsIndex_r3/ROM  depth=256  initVector=sqrt(2) * cos(pi*((0:255) + 0.5)*2^(-8))  arith_type="Signed  (2's comp)"  n_bits=10  bin_pt=8  latency=1  distributed_mem=off  init_zero=on  explicit_period=off  period=1  en=off  dbl_ovrd=off  gen_core=on  use_rpm=off
      settings: xl_area=[0, 0, 0, 0, 0, 0, 0]
  lfsr_47_5 : Subsystem  mask(lfsr_47){init=init}
      mask prompts: init "init(47:1)"
  g(s') : Outport
  wires:
  ROM/1 -> Delay/1
  lfsr_47_5/1(" ") -> ROM/1
  Delay/1 -> g(s')/1
  reset/1 -> lfsr_47_5/1(reset)

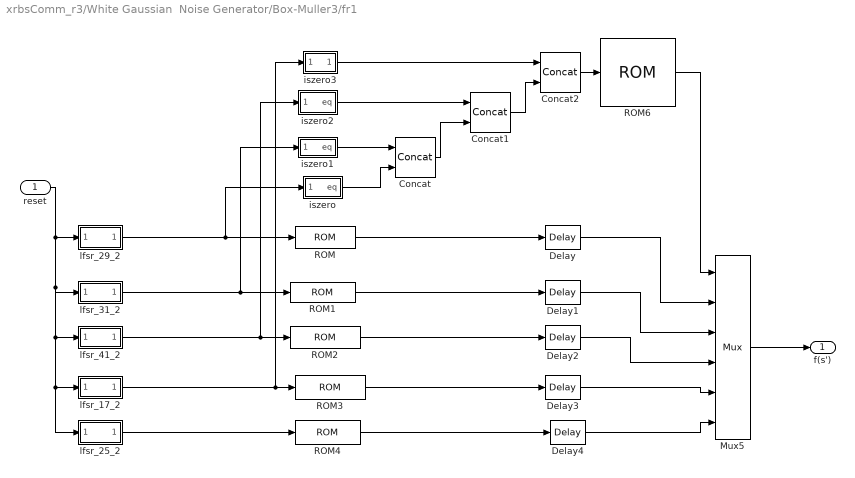
== system xrbsComm_r3/White Gaussian  Noise Generator/Box-Muller3/fr1 ==
  reset : Inport
  Concat : xbsIndex_r3/Concat  explicit_period=off  period=1  dbl_ovrd=off
  Concat1 : xbsIndex_r3/Concat  explicit_period=off  period=1  dbl_ovrd=off
  Concat2 : xbsIndex_r3/Concat  explicit_period=off  period=1  dbl_ovrd=off
  Delay{,1..4} (5 alike) : xbsIndex_r3/Delay  latency=2  explicit_period=off  period=1  en=off  accept_only_valid=off  init_zero=on  dbl_ovrd=off
      settings: xl_area=[0, 0, 0, 0, 0, 0, 0]
  Mux5 : xbsIndex_r3/Mux  inputs=5  precision=Full  arith_type="Signed  (2's comp)"  n_bits=10  bin_pt=0  quantization="Round  (unbiased: +/- Inf)"  overflow=Wrap  latency=1  mux_type=off  explicit_period=off  period=1  en=off  dbl_ovrd=off  gen_core=on  use_rpm=off
      settings: xl_area=[0, 0, 0, 0, 0, 0, 0]
  ROM : xbsIndex_r3/ROM  depth=16  initVector=sqrt(-log( ((0:15)+0.51)'*(2.^(-1.*4)) ))  arith_type=Unsigned  n_bits=9  bin_pt=7  latency=1  distributed_mem=on  init_zero=on  explicit_period=off  period=1  en=off  dbl_ovrd=off  gen_core=on  use_rpm=off
      settings: xl_area=[0, 0, 0, 0, 0, 0, 0]
  ROM1 : xbsIndex_r3/ROM  depth=16  initVector=sqrt(-log( ((0:15)+0.51)'*(2.^(-2.*4)) ))  arith_type=Unsigned  n_bits=9  bin_pt=7  latency=1  distributed_mem=on  init_zero=on  explicit_period=off  period=1  en=off  dbl_ovrd=off  gen_core=on  use_rpm=off
      settings: xl_area=[0, 0, 0, 0, 0, 0, 0]
  ROM2 : xbsIndex_r3/ROM  depth=16  initVector=sqrt(-log( ((0:15)+0.51)'*(2.^(-3.*4)) ))  arith_type=Unsigned  n_bits=9  bin_pt=7  latency=1  distributed_mem=on  init_zero=on  explicit_period=off  period=1  en=off  dbl_ovrd=off  gen_core=on  use_rpm=off
      settings: xl_area=[0, 0, 0, 0, 0, 0, 0]
  ROM3 : xbsIndex_r3/ROM  depth=16  initVector=sqrt(-log( ((0:15)+0.51)'*(2.^(-4.*4)) ))  arith_type=Unsigned  n_bits=9  bin_pt=7  latency=1  distributed_mem=on  init_zero=on  explicit_period=off  period=1  en=off  dbl_ovrd=off  gen_core=on  use_rpm=off
      settings: xl_area=[0, 0, 0, 0, 0, 0, 0]
  ROM4 : xbsIndex_r3/ROM  depth=16  initVector=sqrt(-log( ((0:15)+0.51)'*(2.^(-5.*4)) ))  arith_type=Unsigned  n_bits=9  bin_pt=7  latency=1  distributed_mem=on  init_zero=on  explicit_period=off  period=1  en=off  dbl_ovrd=off  gen_core=on  use_rpm=off
      settings: xl_area=[0, 0, 0, 0, 0, 0, 0]
  ROM6 : xbsIndex_r3/ROM  depth=16  initVector=[0 1 0 2 0 1 0 3 0 1 0 2 0 1 0 4]  arith_type=Unsigned  n_bits=3  bin_pt=0  latency=2  distributed_mem=off  init_zero=on  explicit_period=off  period=1  en=off  dbl_ovrd=off  gen_core=on  use_rpm=off
      settings: xl_area=[0, 0, 0, 0, 0, 0, 0]
  iszero : Subsystem
  iszero1 : Subsystem
  iszero2 : Subsystem
  iszero3 : Subsystem
  lfsr_17_2 : Subsystem  mask(lfsr_17){init=init1}
      mask prompts: init "init(17:1)"
  lfsr_25_2 : Subsystem  mask(lfsr_25){init=init2}
      mask prompts: init "init(25:1)"
  lfsr_29_2 : Subsystem  mask(lfsr_29){init=init3}
      mask prompts: init "init(29:1)"
  lfsr_31_2 : Subsystem  mask(lfsr_31){init=init4}
      mask prompts: init "init(31:1)"
  lfsr_41_2 : Subsystem  mask(lfsr_41){init=init5}
      mask prompts: init "init(41:1)"
  f(s') : Outport
  wires:
  lfsr_29_2/1(" ") -> ROM/1, iszero/1(" ")
  lfsr_31_2/1(" ") -> ROM1/1, iszero1/1(" ")
  lfsr_41_2/1(" ") -> ROM2/1, iszero2/1(" ")
  lfsr_17_2/1(" ") -> iszero3/1(" "), ROM3/1
  lfsr_25_2/1(" ") -> ROM4/1
  Mux5/1 -> f(s')/1
  Concat/1 -> Concat1/2
  Concat1/1 -> Concat2/2
  Concat2/1 -> ROM6/1
  ROM6/1 -> Mux5/1
  ROM/1 -> Delay/1
  ROM1/1 -> Delay1/1
  ROM2/1 -> Delay2/1
  ROM3/1 -> Delay3/1
  ROM4/1 -> Delay4/1
  iszero/1(eq) -> Concat/2
  iszero1/1(eq) -> Concat/1
  iszero2/1(eq) -> Concat1/1
  iszero3/1(eq) -> Concat2/1
  Delay4/1 -> Mux5/6
  Delay3/1 -> Mux5/5
  Delay2/1 -> Mux5/4
  Delay1/1 -> Mux5/3
  Delay/1 -> Mux5/2
  reset/1 -> lfsr_31_2/1(reset), lfsr_41_2/1(reset), lfsr_25_2/1(" reset"), lfsr_17_2/1(reset), lfsr_29_2/1(reset)

== system xrbsComm_r3/White Gaussian  Noise Generator/Box-Muller3/g2 ==
  reset : Inport
  Delay : xbsIndex_r3/Delay  latency=3  explicit_period=off  period=1  en=off  accept_only_valid=off  init_zero=on  dbl_ovrd=off
      settings: xl_area=[0, 0, 0, 0, 0, 0, 0]
  ROM : xbsIndex_r3/ROM  depth=256  initVector=sqrt(2) * cos(pi*((0:255) + 0.5)*2^(-8))  arith_type="Signed  (2's comp)"  n_bits=10  bin_pt=8  latency=1  distributed_mem=off  init_zero=on  explicit_period=off  period=1  en=off  dbl_ovrd=off  gen_core=on  use_rpm=off
      settings: xl_area=[0, 0, 0, 0, 0, 0, 0]
  lfsr_47_5 : Subsystem  mask(lfsr_47){init=init}
      mask prompts: init "init(47:1)"
  g(s') : Outport
  wires:
  ROM/1 -> Delay/1
  Delay/1 -> g(s')/1
  reset/1 -> lfsr_47_5/1(reset)
  lfsr_47_5/1(" ") -> ROM/1

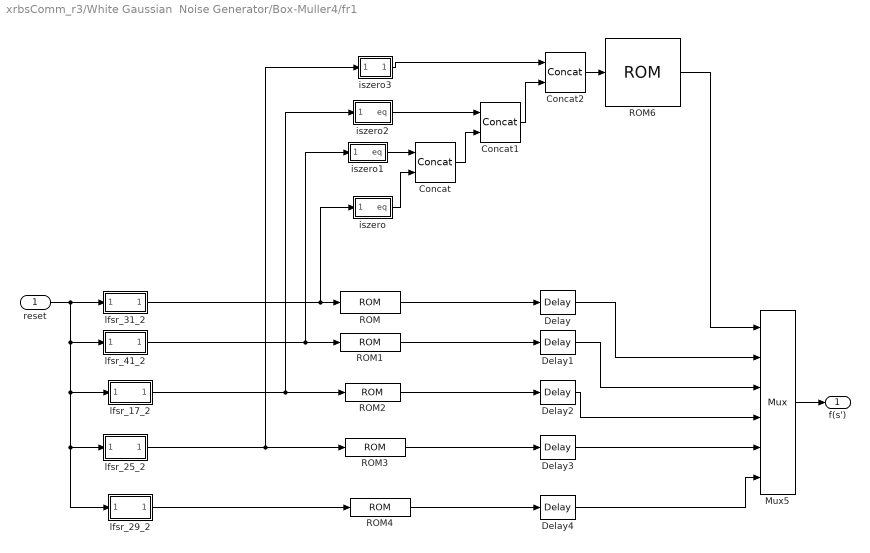
== system xrbsComm_r3/White Gaussian  Noise Generator/Box-Muller4/fr1 ==
  reset : Inport
  Concat : xbsIndex_r3/Concat  explicit_period=off  period=1  dbl_ovrd=off
  Concat1 : xbsIndex_r3/Concat  explicit_period=off  period=1  dbl_ovrd=off
  Concat2 : xbsIndex_r3/Concat  explicit_period=off  period=1  dbl_ovrd=off
  Delay{,1..4} (5 alike) : xbsIndex_r3/Delay  latency=2  explicit_period=off  period=1  en=off  accept_only_valid=off  init_zero=on  dbl_ovrd=off
      settings: xl_area=[0, 0, 0, 0, 0, 0, 0]
  Mux5 : xbsIndex_r3/Mux  inputs=5  precision=Full  arith_type="Signed  (2's comp)"  n_bits=10  bin_pt=0  quantization="Round  (unbiased: +/- Inf)"  overflow=Wrap  latency=1  mux_type=off  explicit_period=off  period=1  en=off  dbl_ovrd=off  gen_core=on  use_rpm=off
      settings: xl_area=[0, 0, 0, 0, 0, 0, 0]
  ROM : xbsIndex_r3/ROM  depth=16  initVector=sqrt(-log( ((0:15)+0.51)'*(2.^(-1.*4)) ))  arith_type=Unsigned  n_bits=9  bin_pt=7  latency=1  distributed_mem=on  init_zero=on  explicit_period=off  period=1  en=off  dbl_ovrd=off  gen_core=on  use_rpm=off
      settings: xl_area=[0, 0, 0, 0, 0, 0, 0]
  ROM1 : xbsIndex_r3/ROM  depth=16  initVector=sqrt(-log( ((0:15)+0.51)'*(2.^(-2.*4)) ))  arith_type=Unsigned  n_bits=9  bin_pt=7  latency=1  distributed_mem=on  init_zero=on  explicit_period=off  period=1  en=off  dbl_ovrd=off  gen_core=on  use_rpm=off
      settings: xl_area=[0, 0, 0, 0, 0, 0, 0]
  ROM2 : xbsIndex_r3/ROM  depth=16  initVector=sqrt(-log( ((0:15)+0.51)'*(2.^(-3.*4)) ))  arith_type=Unsigned  n_bits=9  bin_pt=7  latency=1  distributed_mem=on  init_zero=on  explicit_period=off  period=1  en=off  dbl_ovrd=off  gen_core=on  use_rpm=off
      settings: xl_area=[0, 0, 0, 0, 0, 0, 0]
  ROM3 : xbsIndex_r3/ROM  depth=16  initVector=sqrt(-log( ((0:15)+0.51)'*(2.^(-4.*4)) ))  arith_type=Unsigned  n_bits=9  bin_pt=7  latency=1  distributed_mem=on  init_zero=on  explicit_period=off  period=1  en=off  dbl_ovrd=off  gen_core=on  use_rpm=off
      settings: xl_area=[0, 0, 0, 0, 0, 0, 0]
  ROM4 : xbsIndex_r3/ROM  depth=16  initVector=sqrt(-log( ((0:15)+0.51)'*(2.^(-5.*4)) ))  arith_type=Unsigned  n_bits=9  bin_pt=7  latency=1  distributed_mem=on  init_zero=on  explicit_period=off  period=1  en=off  dbl_ovrd=off  gen_core=on  use_rpm=off
      settings: xl_area=[0, 0, 0, 0, 0, 0, 0]
  ROM6 : xbsIndex_r3/ROM  depth=16  initVector=[0 1 0 2 0 1 0 3 0 1 0 2 0 1 0 4]  arith_type=Unsigned  n_bits=3  bin_pt=0  latency=2  distributed_mem=off  init_zero=on  explicit_period=off  period=1  en=off  dbl_ovrd=off  gen_core=on  use_rpm=off
      settings: xl_area=[0, 0, 0, 0, 0, 0, 0]
  iszero : Subsystem
  iszero1 : Subsystem
  iszero2 : Subsystem
  iszero3 : Subsystem
  lfsr_17_2 : Subsystem  mask(lfsr_17){init=init1}
      mask prompts: init "init(17:1)"
  lfsr_25_2 : Subsystem  mask(lfsr_25){init=init2}
      mask prompts: init "init(25:1)"
  lfsr_29_2 : Subsystem  mask(lfsr_29){init=init3}
      mask prompts: init "init(29:1)"
  lfsr_31_2 : Subsystem  mask(lfsr_31){init=init4}
      mask prompts: init "init(31:1)"
  lfsr_41_2 : Subsystem  mask(lfsr_41){init=init5}
      mask prompts: init "init(41:1)"
  f(s') : Outport
  wires:
  iszero/1(eq) -> Concat/2
  lfsr_31_2/1(" ") -> ROM/1, iszero/1(" ")
  lfsr_41_2/1(" ") -> iszero1/1(" "), ROM1/1
  lfsr_17_2/1(" ") -> ROM2/1, iszero2/1(" ")
  lfsr_25_2/1(" ") -> ROM3/1, iszero3/1(" ")
  ROM6/1 -> Mux5/1
  Concat/1 -> Concat1/2
  Concat1/1 -> Concat2/2
  ROM/1 -> Delay/1
  ROM1/1 -> Delay1/1
  Concat2/1 -> ROM6/1
  ROM2/1 -> Delay2/1
  ROM3/1 -> Delay3/1
  ROM4/1 -> Delay4/1
  iszero1/1(eq) -> Concat/1
  iszero2/1(eq) -> Concat1/1
  iszero3/1(eq) -> Concat2/1
  Mux5/1 -> f(s')/1
  Delay4/1 -> Mux5/6
  Delay3/1 -> Mux5/5
  Delay2/1 -> Mux5/4
  Delay1/1 -> Mux5/3
  Delay/1 -> Mux5/2
  lfsr_29_2/1(" ") -> ROM4/1
  reset/1 -> lfsr_41_2/1(reset), lfsr_17_2/1(reset), lfsr_25_2/1(" reset"), lfsr_29_2/1(reset), lfsr_31_2/1(reset)

== system xrbsComm_r3/White Gaussian  Noise Generator/Box-Muller4/g2 ==
  reset : Inport
  Delay : xbsIndex_r3/Delay  latency=2  explicit_period=off  period=1  en=off  accept_only_valid=off  init_zero=on  dbl_ovrd=off
      settings: xl_area=[0, 0, 0, 0, 0, 0, 0]
  Delay1 : xbsIndex_r3/Delay  latency=1  explicit_period=off  period=1  en=off  accept_only_valid=off  init_zero=on  dbl_ovrd=off
      settings: xl_area=[0, 0, 0, 0, 0, 0, 0]
  ROM : xbsIndex_r3/ROM  depth=256  initVector=sqrt(2) * cos(pi*((0:255) + 0.5)*2^(-8))  arith_type="Signed  (2's comp)"  n_bits=10  bin_pt=8  latency=1  distributed_mem=off  init_zero=on  explicit_period=off  period=1  en=off  dbl_ovrd=off  gen_core=on  use_rpm=off
      settings: xl_area=[0, 0, 0, 0, 0, 0, 0]
  lfsr_47_5 : Subsystem  mask(lfsr_47){init=init}
      mask prompts: init "init(47:1)"
  g(s') : Outport
  wires:
  Delay1/1 -> ROM/1
  ROM/1 -> Delay/1
  lfsr_47_5/1(" ") -> Delay1/1
  Delay/1 -> g(s')/1
  reset/1 -> lfsr_47_5/1(reset)

== system xrbsComm_r3/White Gaussian  Noise Generator/Box-Muller1/f/iszero ==
  " " : Inport
  Constant : xbsIndex_r3/Constant  const=0  arith_type=Unsigned  n_bits=4  bin_pt=0  explicit_period=off  period=1  dbl_ovrd=off
  sel1 : xbsIndex_r3/Relational  mode=a=b  latency=1  explicit_period=off  period=1  en=off  dbl_ovrd=off
      settings: xl_area=[0, 0, 0, 0, 0, 0, 0]
  eq : Outport
  wires:
  Constant/1 -> sel1/2
  " "/1 -> sel1/1
  sel1/1 -> eq/1

== system xrbsComm_r3/White Gaussian  Noise Generator/Box-Muller1/f/iszero1 ==
  " " : Inport
  Constant : xbsIndex_r3/Constant  const=0  arith_type=Unsigned  n_bits=4  bin_pt=0  explicit_period=off  period=1  dbl_ovrd=off
  sel2 : xbsIndex_r3/Relational  mode=a=b  latency=1  explicit_period=off  period=1  en=off  dbl_ovrd=off
      settings: xl_area=[0, 0, 0, 0, 0, 0, 0]
  eq : Outport
  wires:
  Constant/1 -> sel2/2
  " "/1 -> sel2/1
  sel2/1 -> eq/1

== system xrbsComm_r3/White Gaussian  Noise Generator/Box-Muller1/f/iszero2 ==
  " " : Inport
  Constant : xbsIndex_r3/Constant  const=0  arith_type=Unsigned  n_bits=4  bin_pt=0  explicit_period=off  period=1  dbl_ovrd=off
  sel3 : xbsIndex_r3/Relational  mode=a=b  latency=1  explicit_period=off  period=1  en=off  dbl_ovrd=off
      settings: xl_area=[0, 0, 0, 0, 0, 0, 0]
  eq : Outport
  wires:
  Constant/1 -> sel3/2
  " "/1 -> sel3/1
  sel3/1 -> eq/1

== system xrbsComm_r3/White Gaussian  Noise Generator/Box-Muller1/f/iszero3 ==
  " " : Inport
  Constant : xbsIndex_r3/Constant  const=0  arith_type=Unsigned  n_bits=4  bin_pt=0  explicit_period=off  period=1  dbl_ovrd=off
  sel4 : xbsIndex_r3/Relational  mode=a=b  latency=1  explicit_period=off  period=1  en=off  dbl_ovrd=off
      settings: xl_area=[0, 0, 0, 0, 0, 0, 0]
  eq : Outport
  wires:
  Constant/1 -> sel4/2
  " "/1 -> sel4/1
  sel4/1 -> eq/1

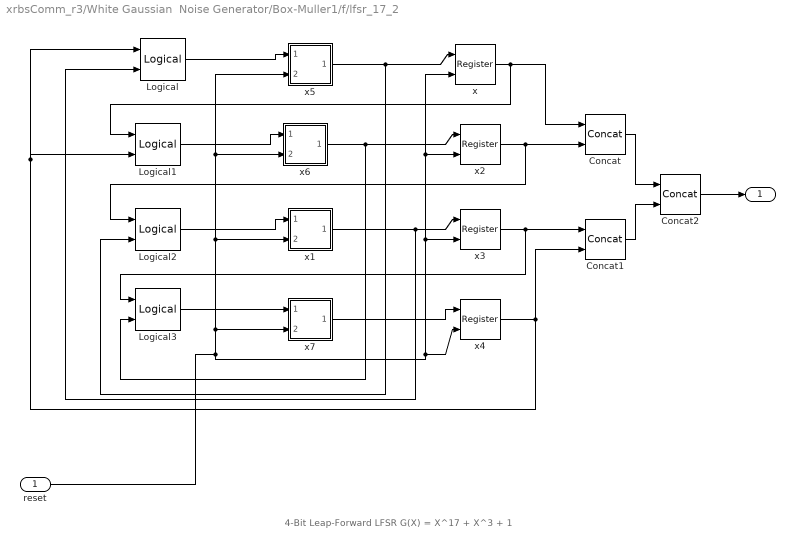
== system xrbsComm_r3/White Gaussian  Noise Generator/Box-Muller1/f/lfsr_17_2 ==
  note: 4-Bit Leap-Forward LFSR G(X) = X^17 + X^3 + 1
  reset : Inport
  Concat : xbsIndex_r3/Concat  explicit_period=off  period=1  dbl_ovrd=off
  Concat1 : xbsIndex_r3/Concat  explicit_period=off  period=1  dbl_ovrd=off
  Concat2 : xbsIndex_r3/Concat  explicit_period=off  period=1  dbl_ovrd=off
  Logical{,1..3} (4 alike) : xbsIndex_r3/Logical  logical_function=XOR  inputs=2  precision=User Defined  arith_type=Unsigned  n_bits=1  bin_pt=0  align_bp=on  latency=0  explicit_period=on  period=-1  en=off  dbl_ovrd=off
      settings: xl_area=[0, 0, 0, 0, 0, 0, 0]
  x : xbsIndex_r3/Register  init=init(1)  reg_only_valid=off  explicit_period=off  period=1  rst=on  en=off  out_en=off  dbl_ovrd=off
      settings: xl_area=[0, 0, 0, 0, 0, 0, 0]
  x1 : Subsystem  mask{init=init(7:4:15)}
  x2 : xbsIndex_r3/Register  init=init(2)  reg_only_valid=off  explicit_period=off  period=1  rst=on  en=off  out_en=off  dbl_ovrd=off
      settings: xl_area=[0, 0, 0, 0, 0, 0, 0]
  x3 : xbsIndex_r3/Register  init=init(3)  reg_only_valid=off  explicit_period=off  period=1  rst=on  en=off  out_en=off  dbl_ovrd=off
      settings: xl_area=[0, 0, 0, 0, 0, 0, 0]
  x4 : xbsIndex_r3/Register  init=init(4)  reg_only_valid=off  explicit_period=off  period=1  rst=on  en=off  out_en=off  dbl_ovrd=off
      settings: xl_area=[0, 0, 0, 0, 0, 0, 0]
  x5 : Subsystem  mask{init=init(5:4:17)}
  x6 : Subsystem  mask{init=init(6:4:14)}
  x7 : Subsystem  mask{init=init(8:4:16)}
  " " : Outport
  wires:
  Logical/1 -> x5/1(" ")
  Logical1/1 -> x6/1(" ")
  Logical2/1 -> x1/1(" ")
  Logical3/1 -> x7/1(" ")
  x5/1(z-4) -> x/1, Logical2/2
  x6/1(z-3) -> x2/1, Logical3/2
  x1/1(z-3) -> x3/1, Logical/2
  x7/1(z-3) -> x4/1
  x/1 -> Concat/1, Logical1/1
  x2/1 -> Concat/2, Logical2/1
  Concat/1 -> Concat2/1
  x3/1 -> Concat1/1, Logical3/1
  x4/1 -> Concat1/2, Logical1/2, Logical/1
  Concat1/1 -> Concat2/2
  Concat2/1 -> " "/1
  reset/1 -> x5/2(reset), x6/2(" reset"), x1/2(" reset"), x7/2(reset), x/2, x2/2, x3/2, x4/2

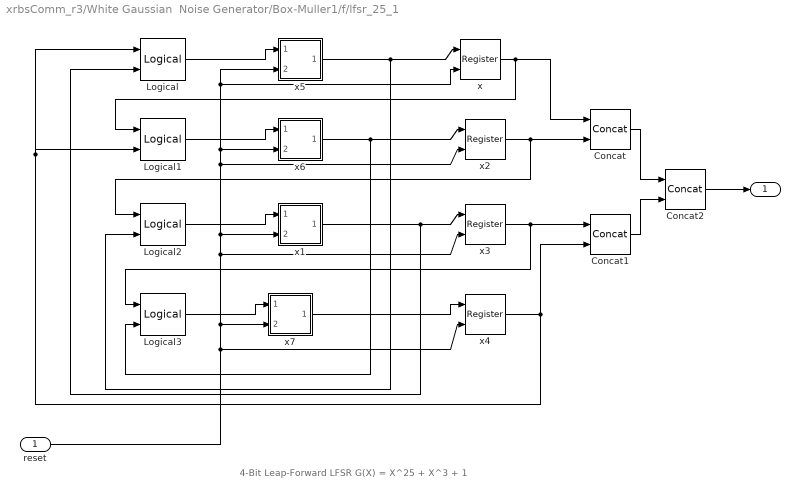
== system xrbsComm_r3/White Gaussian  Noise Generator/Box-Muller1/f/lfsr_25_1 ==
  note: 4-Bit Leap-Forward LFSR G(X) = X^25 + X^3 + 1
  " reset" : Inport
  Concat : xbsIndex_r3/Concat  explicit_period=off  period=1  dbl_ovrd=off
  Concat1 : xbsIndex_r3/Concat  explicit_period=off  period=1  dbl_ovrd=off
  Concat2 : xbsIndex_r3/Concat  explicit_period=off  period=1  dbl_ovrd=off
  Logical{,1..3} (4 alike) : xbsIndex_r3/Logical  logical_function=XOR  inputs=2  precision=User Defined  arith_type=Unsigned  n_bits=1  bin_pt=0  align_bp=on  latency=0  explicit_period=on  period=-1  en=off  dbl_ovrd=off
      settings: xl_area=[0, 0, 0, 0, 0, 0, 0]
  x : xbsIndex_r3/Register  init=init(1)  reg_only_valid=off  explicit_period=off  period=1  rst=on  en=off  out_en=off  dbl_ovrd=off
      settings: xl_area=[0, 0, 0, 0, 0, 0, 0]
  x1 : Subsystem  mask{init=init(7:4:23)}
  x2 : xbsIndex_r3/Register  init=init(2)  reg_only_valid=off  explicit_period=off  period=1  rst=on  en=off  out_en=off  dbl_ovrd=off
      settings: xl_area=[0, 0, 0, 0, 0, 0, 0]
  x3 : xbsIndex_r3/Register  init=init(3)  reg_only_valid=off  explicit_period=off  period=1  rst=on  en=off  out_en=off  dbl_ovrd=off
      settings: xl_area=[0, 0, 0, 0, 0, 0, 0]
  x4 : xbsIndex_r3/Register  init=init(4)  reg_only_valid=off  explicit_period=off  period=1  rst=on  en=off  out_en=off  dbl_ovrd=off
      settings: xl_area=[0, 0, 0, 0, 0, 0, 0]
  x5 : Subsystem  mask{init=init(5:4:25)}
  x6 : Subsystem  mask{init=init(6:4:22)}
  x7 : Subsystem  mask{init=init(8:4:24)}
  " " : Outport
  wires:
  Concat2/1 -> " "/1
  Concat1/1 -> Concat2/2
  x4/1 -> Logical/1, Logical1/2, Concat1/2
  x3/1 -> Logical3/1, Concat1/1
  Concat/1 -> Concat2/1
  x2/1 -> Logical2/1, Concat/2
  x/1 -> Concat/1, Logical1/1
  x7/1(z-5) -> x4/1
  x1/1(z-5) -> Logical/2, x3/1
  x6/1(z-5) -> Logical3/2, x2/1
  x5/1(z-6) -> Logical2/2, x/1
  Logical3/1 -> x7/1(" ")
  Logical2/1 -> x1/1(" ")
  Logical1/1 -> x6/1(" ")
  Logical/1 -> x5/1(" ")
  " reset"/1 -> x7/2(reset), x1/2(reset), x6/2(reset), x5/2(reset), x/2, x2/2, x3/2, x4/2

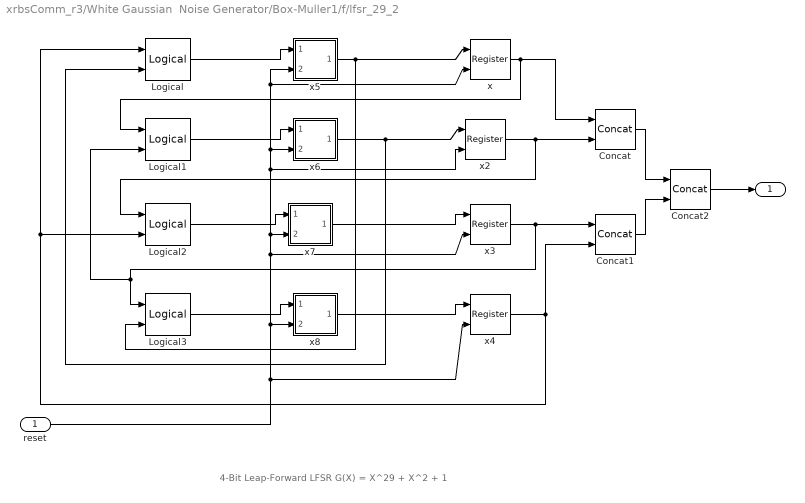
== system xrbsComm_r3/White Gaussian  Noise Generator/Box-Muller1/f/lfsr_29_2 ==
  note: 4-Bit Leap-Forward LFSR G(X) = X^29 + X^2 + 1
  reset : Inport
  Concat : xbsIndex_r3/Concat  explicit_period=off  period=1  dbl_ovrd=off
  Concat1 : xbsIndex_r3/Concat  explicit_period=off  period=1  dbl_ovrd=off
  Concat2 : xbsIndex_r3/Concat  explicit_period=off  period=1  dbl_ovrd=off
  Logical{,1..3} (4 alike) : xbsIndex_r3/Logical  logical_function=XOR  inputs=2  precision=User Defined  arith_type=Unsigned  n_bits=1  bin_pt=0  align_bp=on  latency=0  explicit_period=on  period=-1  en=off  dbl_ovrd=off
      settings: xl_area=[0, 0, 0, 0, 0, 0, 0]
  x : xbsIndex_r3/Register  init=init(1)  reg_only_valid=off  explicit_period=off  period=1  rst=on  en=off  out_en=off  dbl_ovrd=off
      settings: xl_area=[0, 0, 0, 0, 0, 0, 0]
  x2 : xbsIndex_r3/Register  init=init(2)  reg_only_valid=off  explicit_period=off  period=1  rst=on  en=off  out_en=off  dbl_ovrd=off
      settings: xl_area=[0, 0, 0, 0, 0, 0, 0]
  x3 : xbsIndex_r3/Register  init=init(3)  reg_only_valid=off  explicit_period=off  period=1  rst=on  en=off  out_en=off  dbl_ovrd=off
      settings: xl_area=[0, 0, 0, 0, 0, 0, 0]
  x4 : xbsIndex_r3/Register  init=init(4)  reg_only_valid=off  explicit_period=off  period=1  rst=on  en=off  out_en=off  dbl_ovrd=off
      settings: xl_area=[0, 0, 0, 0, 0, 0, 0]
  x5 : Subsystem  mask{init=init(5:4:29)}
  x6 : Subsystem  mask{init=init(6:4:26)}
  x7 : Subsystem  mask{init=init(7:4:27)}
  x8 : Subsystem  mask{init=init(8:4:28)}
  " " : Outport
  wires:
  Logical/1 -> x5/1(" ")
  Logical1/1 -> x6/1(" ")
  Logical2/1 -> x7/1(" ")
  Logical3/1 -> x8/1(" ")
  x5/1(z-7) -> x/1, Logical3/2
  x6/1(z-6) -> x2/1, Logical/2
  x7/1(z-6) -> x3/1
  x8/1(z-6) -> x4/1
  x/1 -> Logical1/1, Concat/1
  x2/1 -> Concat/2, Logical2/1
  Concat/1 -> Concat2/1
  x3/1 -> Concat1/1, Logical3/1, Logical1/2
  x4/1 -> Concat1/2, Logical2/2, Logical/1
  Concat1/1 -> Concat2/2
  Concat2/1 -> " "/1
  reset/1 -> x8/2(reset), x7/2(reset), x6/2(reset), x5/2(reset), x/2, x2/2, x3/2, x4/2

== system xrbsComm_r3/White Gaussian  Noise Generator/Box-Muller1/f/lfsr_31_2 ==
  note: 4-Bit Leap-Forward LFSR G(X) = X^31 + X^3 + 1
  reset : Inport
  Concat : xbsIndex_r3/Concat  explicit_period=off  period=1  dbl_ovrd=off
  Concat1 : xbsIndex_r3/Concat  explicit_period=off  period=1  dbl_ovrd=off
  Concat2 : xbsIndex_r3/Concat  explicit_period=off  period=1  dbl_ovrd=off
  Logical{,1..3} (4 alike) : xbsIndex_r3/Logical  logical_function=XOR  inputs=2  precision=User Defined  arith_type=Unsigned  n_bits=1  bin_pt=0  align_bp=on  latency=0  explicit_period=on  period=-1  en=off  dbl_ovrd=off
      settings: xl_area=[0, 0, 0, 0, 0, 0, 0]
  x : xbsIndex_r3/Register  init=init(1)  reg_only_valid=off  explicit_period=off  period=1  rst=on  en=off  out_en=off  dbl_ovrd=off
      settings: xl_area=[0, 0, 0, 0, 0, 0, 0]
  x2 : xbsIndex_r3/Register  init=init(2)  reg_only_valid=off  explicit_period=off  period=1  rst=on  en=off  out_en=off  dbl_ovrd=off
      settings: xl_area=[0, 0, 0, 0, 0, 0, 0]
  x3 : xbsIndex_r3/Register  init=init(3)  reg_only_valid=off  explicit_period=off  period=1  rst=on  en=off  out_en=off  dbl_ovrd=off
      settings: xl_area=[0, 0, 0, 0, 0, 0, 0]
  x4 : xbsIndex_r3/Register  init=init(4)  reg_only_valid=off  explicit_period=off  period=1  rst=on  en=off  out_en=off  dbl_ovrd=off
      settings: xl_area=[0, 0, 0, 0, 0, 0, 0]
  x5 : Subsystem  mask{init=init(5:4:29)}
  x6 : Subsystem  mask{init=init(6:4:30)}
  x7 : Subsystem  mask{init=init(7:4:31)}
  x8 : Subsystem  mask{init=init(8:4:28)}
  " " : Outport
  wires:
  Logical/1 -> x5/1(" ")
  Logical1/1 -> x6/1(" ")
  Logical2/1 -> x7/1(" ")
  Logical3/1 -> x8/1(" ")
  x5/1(z-7) -> Logical/1, x/1
  x6/1(z-7) -> Logical1/1, x2/1
  x7/1(z-7) -> x3/1, Logical2/1
  x8/1(z-6) -> x4/1
  x/1 -> Concat/1, Logical3/1
  x2/1 -> Concat/2, Logical/2
  Concat/1 -> Concat2/1
  x3/1 -> Concat1/1, Logical1/2
  x4/1 -> Logical2/2, Concat1/2, Logical3/2
  Concat1/1 -> Concat2/2
  Concat2/1 -> " "/1
  reset/1 -> x5/2(reset), x6/2(reset), x7/2(reset), x8/2(reset), x/2, x2/2, x3/2, x4/2
